simulink model "DZ_DSMC"  (R2020a)
settings: Solver=FixedStepAuto  StartTime=0.0  StopTime=30  FixedStep=Ts  MaxStep=0.015  RelTol=1e-3
PreLoadFcn:
  | if ~exist('sim_HIL')
  |     sim_HIL=false;
  | end
  | if ~exist('usefilter')
  |     usefilter=false;
  | end
InitFcn:
  | load motorModel.mat
  | load expsetup
model workspace (MAT data in the model file):
  C = [5000.03981444; 99.8743032511]
  N = 10
  del = 0.190672986837
  eta = 1
  gamm = 10
  nodeID = 2
  qT = 0.0615444828285
  vphi = 1.00000000056
  xiT = 0.997380636587
values from neighbouring files (symbols this model uses):
  Ts = 0.015    [ParamSetup.m]    (also in motorModel.mat = 0.002)
undefined symbols (not defined in the file or in its folder): mModel, x607325_PPR
undefined symbols (not defined in the file): k, X
libraries: simulink x1
settings Model: DataDictionary=MotorInfo.sldd  Creator=khoi  LastModifiedBy=khoi
settings DataIOCC: SaveOutput=off  SaveTime=off
settings OptimizationCC: DefaultParameterBehavior=Inlined  UseDivisionForNetSlopeComputation=on  GainParamInheritBuiltInType=on  UseFloatMulNetSlope=on  UseSpecifiedMinMax=on  InlineInvariantSignals=on  BitwiseOrLogicalOp=Bitwise operator  PassReuseOutputArgsAs=Individual arguments  ZeroExternalMemoryAtStartup=off  ZeroInternalMemoryAtStartup=off  NoFixptDivByZeroProtection=on  EfficientFloat2IntCast=on  LifeSpan=1  OptimizeBlockOrder=speed  DifferentSizesBufferReuse=on  EfficientTunableParamExpr=on
settings DebuggingCC: AlgebraicLoopMsg=none  ParameterTunabilityLossMsg=error
settings HardwareCC: ProdLongLongMode=on
settings SFSimCC: MATLABDynamicMemAlloc=off
settings RTWCC: SystemTargetFile=ert.tlc  TemplateMakefile=ert_default_tmf  GenerateReport=on  BuildConfiguration=Faster Runs  LaunchReport=on
settings CodeAppCC: ForceParamTrailComments=on  IgnoreCustomStorageClasses=off  OperatorAnnotations=on  SimulinkDataObjDesc=on  SFDataObjDesc=on  CustomSymbolStrGlobalVar=rt$N$M  CustomSymbolStrType=$N$M  CustomSymbolStrFcn=$N$M$F  CustomSymbolStrMacro=$N$M  InsertBlockDesc=on
settings ERTTargetCC: TargetLangStandard=C99 (ISO)  UtilityFuncGeneration=Shared location  GenerateSampleERTMain=on  IncludeMdlTerminateFcn=off  CombineSignalStateStructs=on  SuppressErrorStatus=on  MultiInstanceERTCode=on  CodeInterfacePackaging=Reusable function  SupportNonFinite=off  SupportComplex=off  InlinedParameterPlacement=NonHierarchical  ERTCustomFileTemplate=example_file_process.tlc  ERTFilePackagingFormat=CompactWithDataFile

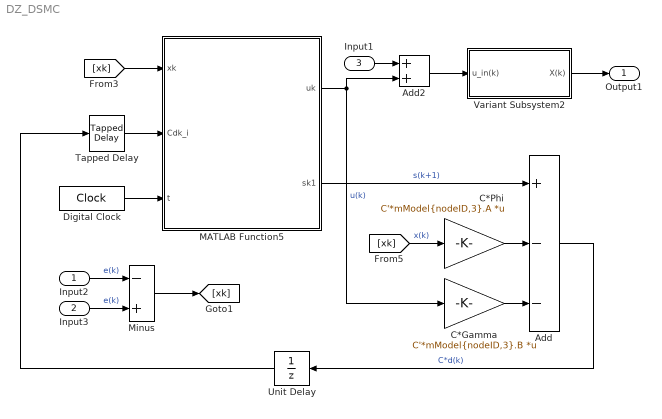
== system DZ_DSMC ==
  Input2 : Inport  PortDimensions=2
  Input3 : Inport  Port=2  PortDimensions=2
  Input1 : Inport  Port=3
  Add : Sum  Inputs=+--
  Add2 : Sum
  C*Gamma : Gain  Gain=C'*mModel{nodeID,3}.B  Multiplication=Matrix(K*u)
  C*Phi : Gain  Gain=C'*mModel{nodeID,3}.A  Multiplication=Matrix(K*u) (u vector)
  Digital Clock : DigitalClock  SampleTime=Ts
  MATLAB Function5 : MATLAB Function  TreatAsAtomicUnit=on  mask{Phi=mModel{nodeID,3}.A, Gam=mModel{nodeID,3}.B, C=C', qT=qT, xiT=xiT, del=del, vphi=vphi, gamm=gamm, eta=eta, Ts=Ts, n=N}
      mask prompts: del "delta"; gamm "gamma"
  Minus : Sum  Inputs=-+
  Tapped Delay : simulink/Discrete/Tapped Delay  vinit=0.0  samptime=-1  NumDelays=N  DelayOrder=Newest  includeCurrent=on
  Unit Delay : UnitDelay  SampleTime=-1  HasFrameUpgradeWarning=on
  Variant Subsystem2 : Subsystem  Variant=on  mask{ss_sys=mModel{nodeID,3}, NodeID=nodeID, Ts=Ts}
      mask prompts: ss_sys "state space model"; NodeID "node ID"; Ts "Sample time (s)"
      mask init:
      | myDictionaryObj = Simulink.data.dictionary.open('MotorInfo.sldd');
      mask DialogControl ParameterGroupVar Prompt: Mathematical model
      mask DialogControl ParameterGroupVar_copy Prompt: Mathematical model
  Output1 : Outport  PortDimensions=2
  wires:
  Unit Delay/1 -> Tapped Delay/1
  Minus/1 -> [xk]
  Input2/1 -> Minus/1  "e(k)"
  Add/1 -> Unit Delay/1  "C*d(k)"
  MATLAB Function5/1(uk) -> Add2/2, C*Gamma/1  "u(k)"
  [xk] -> MATLAB Function5/1(xk)
  [xk] -> C*Phi/1  "x(k)"
  Variant Subsystem2/1(X(k)) -> Output1/1
  Input3/1 -> Minus/2  "e(k)"
  MATLAB Function5/2(sk1) -> Add/1  "s(k+1)"
  C*Gamma/1 -> Add/3
  C*Phi/1 -> Add/2
  Tapped Delay/1 -> MATLAB Function5/2(Cdk_i)
  Add2/1 -> Variant Subsystem2/1(u_in(k))
  Input1/1 -> Add2/1
  Digital Clock/1 -> MATLAB Function5/3(t)

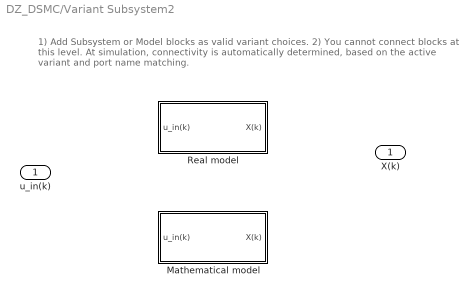
== system DZ_DSMC/Variant Subsystem2 ==
  note: 1) Add Subsystem or Model blocks as valid variant choices.
      | 2) You cannot connect blocks at this level. At simulation, connectivity is automatically
      | determined, based on the active variant and port name matching.
  u_in(k) : Inport
  Mathematical model : Subsystem  VariantControl=sim_HIL == false
  Real model : Subsystem  VariantControl=sim_HIL == true
  X(k) : Outport

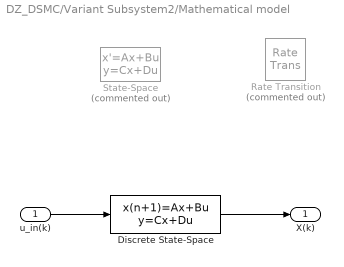
== system DZ_DSMC/Variant Subsystem2/Mathematical model ==
  u_in(k) : Inport
  Discrete State-Space : DiscreteStateSpace  A=ss_sys.A  B=ss_sys.B  C=eye(2)  D=[0;0]  SampleTime=-1
  Rate Transition : RateTransition  Commented=on  OutPortSampleTime=Ts
  State-Space : StateSpace  Commented=on  A=ss_sys.A  B=ss_sys.B  C=eye(2)  D=[0;0]  InitialCondition=0
  X(k) : Outport
  wires:
  Discrete State-Space/1 -> X(k)/1
  u_in(k)/1 -> Discrete State-Space/1

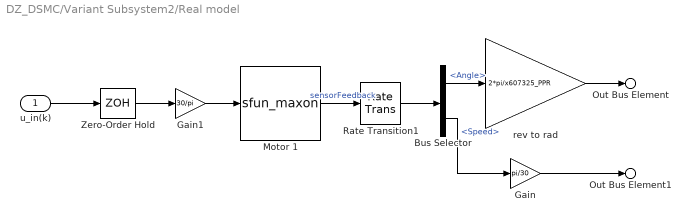
== system DZ_DSMC/Variant Subsystem2/Real model ==
  u_in(k) : Inport
  Bus Selector : BusSelector  OutputSignals=Angle,Speed
  Gain : Gain  Gain=pi/30
  Gain1 : Gain  Gain=30/pi
  Motor 1 : S-Function  FunctionName=sfun_maxon  Parameters=NodeID, DeltaT, OpMode  SFunctionDeploymentMode=off  EnableBusSupport=off  mask{NodeID=NodeID, DeltaT=Ts, OpMode=Cyclic synchronous velocity mode, P_cur=0, I_cur=0, P_pos=0, I_pos=0, D_pos=0, v_posGainFF=0, a_posGainFF=0, P_vel=0, I_vel=0, v_velGainFF=0, a_velGainFF=0, f_velCutoff=0}
      mask prompts: NodeID "Node ID"; DeltaT "Sample time (s)"; OpMode "Operation mode"; P_cur "P gain"; I_cur "I gain"; P_pos "P gain"; I_pos "I gain"; D_pos "D gain"; v_posGainFF "FF velocity gain"; a_posGainFF "FF acceleration gain"; P_vel "P gain"; I_vel "I gain"; v_velGainFF "Feed-forward velocity gain"; a_velGainFF "Feed-forward acceleration gain"; f_velCutoff "Filter cut-off frequency"
      mask TypeOptions OpMode: Cyclic synchronous current (torque) mode | Cyclic synchronous velocity mode | Cyclic synchronous position mode | Profile velocity mode | Profile position mode
      mask DialogControl DescGroupVar Prompt: Motor Parameters
      mask DialogControl DescTextVar Prompt: The block outputs MotorInfo bus signal, which consists of the following variables: angle (increment), speed (rpm), current (mA)
      mask DialogControl Container6 Prompt: Motor
      mask DialogControl Container14 Prompt: Controller Parameters
      mask DialogControl DescTextVar_copy Prompt: This tab is experimental and does not implemented yet. Changing these parameters will not affect the motor performance.
      mask DialogControl Container15 Prompt: Current controller parameter set
      mask DialogControl Container15_copy Prompt: Position controller parameter set
      mask DialogControl Container15_copy_copy Prompt: Velocity controller parameter set
      mask Display:
      | disp('Maxon motor\nHIL');
      | % port_label('input', 1, 'inputSignal');
      | % port_label('output', 1, 'SENSR');
  Rate Transition1 : RateTransition
  Zero-Order Hold : ZeroOrderHold  SampleTime=-1
  rev to rad : Gain  Gain=2*pi/x607325_PPR
  Out Bus Element : Outport  PortName=X(k)  Element=x
  Out Bus Element1 : Outport  PortName=X(k)  Element=dx
  wires:
  Bus Selector/2 -> Gain/1  "<Speed>"
  Bus Selector/1 -> rev to rad/1  "<Angle>"
  Gain1/1 -> Motor 1/1
  rev to rad/1 -> Out Bus Element/1
  Motor 1/1 -> Rate Transition1/1  "sensorFeedback"
  Rate Transition1/1 -> Bus Selector/1
  Zero-Order Hold/1 -> Gain1/1
  u_in(k)/1 -> Zero-Order Hold/1
  Gain/1 -> Out Bus Element1/1

== matlab function DZ_DSMC/MATLAB Function5 ==
  data: xk input; uk output; Cdk_i input; t input; Phi parameter; Gam parameter; C parameter; qT parameter; xiT parameter; del parameter; eta parameter; gamm parameter; vphi parameter; sk1 output; n parameter; Ts parameter
function [uk,sk1] = DeadZoneReachingLaw(xk,Cdk_i,t,...
    Phi, Gam, C, qT, xiT, del, eta, gamm, vphi, n, Ts)

% calcualte switching function
sk = C*xk;

% calculate finite number function
persistent k;
if isempty(k)
    k=0;
end
if rem(t,Ts)==0 && t~=0 && k<n
    k = k+1;
end
vthe = k;

% calculate ud(k) - high-order compensator
udk = 0;
for i=1:vthe
    udk = udk - (-1)^i*nchoosek(vthe,i)*Cdk_i(i+1);
end

% calculate Lambda(k) - exponential function
Lamk= del + (1-del)*exp(-vphi*abs(sk)^gamm);

% calculate rho[s(k)] - dead zone function
if sk>eta
        rhosk=1;
    elseif abs(sk)<=eta
        rhosk=0;
    else % sk<-eta
        rhosk=-1;
end

% calcualte high-order difference function
hodf = Cdk_i(1) - udk;

% calculate one-step forward switching function
sk1 = (1-qT)*Lamk*sk - xiT/Lamk*rhosk + hodf;

% calculate dead zone reaching law controller
uk = -(C*Gam)\(C*Phi*xk - (1-qT)*Lamk*sk + xiT/Lamk*rhosk + udk);
